simulink model "simulacao_com_referencia"  (R2020a)
settings: Solver=ode23s  StartTime=0.0  StopTime=15  FixedStep=0.001  RelTol=1e-3
values from neighbouring files (symbols this model uses):
  C_i = [C 0]    [trabalho_final.m]
  delta = mb*L*L + Ib    (= 0.00848237644)    [trabalho_final.m]
  g = 9.81    [trabalho_final.m]
  gama_i = [gama; 0]    [trabalho_final.m]
  gamah = mb*L    (= 0.039903)    [trabalho_final.m]
  K = place(phi, gama, polos)    [trabalho_final.m]
  Kec_i = inv(phi_i)*Kep_i    [trabalho_final.m]
  Nu = calc(n+1 , 1)    [trabalho_final.m]
  Nx = calc(1:n , 1)    [trabalho_final.m]
  phi_i = [phi gama; zeros(1,n) 1]    [trabalho_final.m]
  Ta = 2*pi/ws    [trabalho_final.m]
settings Model: Creator=arthu  LastModifiedBy=Acer
settings DataIOCC: LimitDataPoints=on  SaveFormat=Array  ReturnWorkspaceOutputs=off
settings OptimizationCC: LifeSpan=inf
settings DebuggingCC: SFUnexpectedBacktrackingDiag=warning  SFNoUnconditionalDefaultTransitionDiag=warning  SFExecutionAtInitializationDiag=none  ArithmeticOperatorsInVariantConditions=warning
settings HardwareCC: ProdBitPerPointer=32  ProdBitPerSizeT=32  ProdBitPerPtrDiffT=32  ProdLargestAtomicFloat=None  ProdIntDivRoundTo=Undefined  ProdEndianess=Unspecified  ProdWordSize=32  ProdHWDeviceType=32-bit Generic
settings ModelReferenceCC: PropagateSignalLabelsOutOfModel=off
settings SFSimCC: SimUseLocalCustomCode=off  CustomCodeUndefinedFunction=UseInterfaceOnly
settings RTWCC: RTWUseLocalCustomCode=off
settings CodeAppCC: StateflowObjectComments=on
settings GRTTargetCC: TargetLangStandard=C89/C90 (ANSI)
settings ConfigComp: CovMetricSettings=dw  CovHtmlReporting=on  CovSaveCumulativeToWorkspaceVar=on  CovSaveSingleToWorkspaceVar=on  CovExternalEMLEnable=off

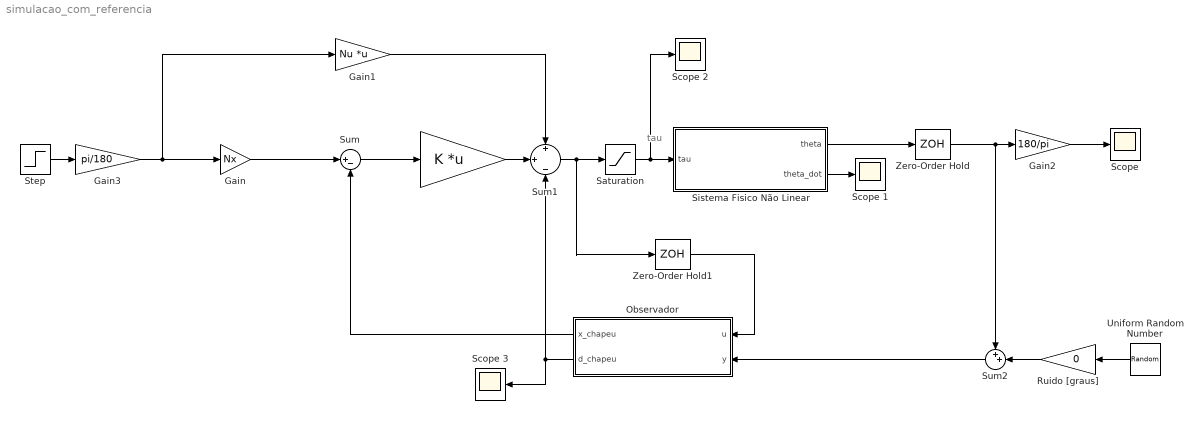
== system simulacao_com_referencia ==
  note: tau
  " " : Gain  Gain=K  Multiplication=Matrix(K*u)
  Gain : Gain  Gain=Nx
  Gain1 : Gain  Gain=Nu  Multiplication=Matrix(K*u)
  Gain2 : Gain  Gain=180/pi
  Gain3 : Gain  Gain=pi/180
  Observador : Subsystem
  Ruido [graus] : Gain  Gain=0
  "Saturation " : Saturate  UpperLimit=0.4118793  LowerLimit=-0.4118793
  Scope {,1..3} (4 alike) : Scope
  Sistema Fisico Não Linear : Subsystem
  Step : Step  After=10  SampleTime=0
  Sum : Sum  Inputs=|+-
  Sum1 : Sum  Inputs=+|+|-
  Sum2 : Sum  Inputs=++|
  "Uniform Random Number " : UniformRandomNumber  Minimum=-pi/180  Maximum=pi/180  SampleTime=Ta
  Zero-Order Hold : ZeroOrderHold  SampleTime=Ta
  Zero-Order Hold1 : ZeroOrderHold  SampleTime=Ta
  wires:
  Sistema Fisico Não Linear/1(theta) -> Zero-Order Hold/1
  Gain2/1 -> "Scope "/1
  Sistema Fisico Não Linear/2(theta_dot) -> Scope 1/1
  Observador/1(x_chapeu) -> Sum/2
  Sum/1 -> " "/1
  Gain/1 -> Sum/1
  Sum1/1 -> Zero-Order Hold1/1, "Saturation "/1
  Gain1/1 -> Sum1/1
  Step/1 -> Gain3/1
  Gain3/1 -> Gain1/1, Gain/1
  "Saturation "/1 -> Sistema Fisico Não Linear/1(tau), Scope 2/1
  Zero-Order Hold/1 -> Sum2/1, Gain2/1
  "Uniform Random Number "/1 -> Ruido [graus]/1
  Ruido [graus]/1 -> Sum2/2
  Observador/2(d_chapeu) -> Scope 3/1, Sum1/3
  " "/1 -> Sum1/2
  Zero-Order Hold1/1 -> Observador/1(u)
  Sum2/1 -> Observador/2(y)

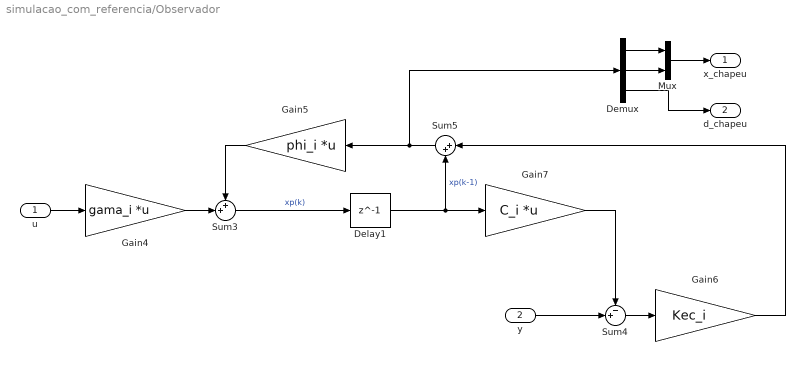
== system simulacao_com_referencia/Observador ==
  u : Inport
  y : Inport  Port=2
  Delay1 : Delay  DelayLength=1  InitialCondition=[0;0;0]
  Demux : Demux  Outputs=3
  Gain4 : Gain  Gain=gama_i  Multiplication=Matrix(K*u) (u vector)
  Gain5 : Gain  Gain=phi_i  Multiplication=Matrix(K*u) (u vector)
  Gain6 : Gain  Gain=Kec_i
  Gain7 : Gain  Gain=C_i  Multiplication=Matrix(K*u) (u vector)
  Mux : Mux  Inputs=2
  Sum3 : Sum  Inputs=++|
  Sum4 : Sum  Inputs=-+|
  Sum5 : Sum  Inputs=|++
  x_chapeu : Outport  VectorParamsAs1DForOutWhenUnconnected=off
  d_chapeu : Outport  Port=2  VectorParamsAs1DForOutWhenUnconnected=off
  wires:
  Gain6/1 -> Sum5/1
  Sum3/1 -> Delay1/1  "xp(k)"
  u/1 -> Gain4/1
  Gain4/1 -> Sum3/2
  Delay1/1 -> Gain7/1, Sum5/2  "xp(k-1)"
  Gain5/1 -> Sum3/1
  Sum4/1 -> Gain6/1
  Gain7/1 -> Sum4/1
  y/1 -> Sum4/2
  Sum5/1 -> Demux/1, Gain5/1
  Mux/1 -> x_chapeu/1
  Demux/1 -> Mux/1
  Demux/2 -> Mux/2
  Demux/3 -> d_chapeu/1

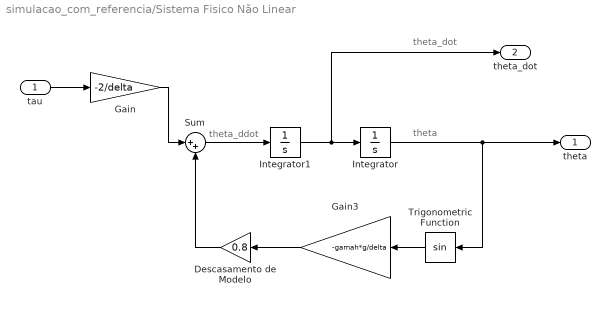
== system simulacao_com_referencia/Sistema Fisico Não Linear ==
  note: theta
  note: theta_dot
  note: theta_ddot
  tau : Inport
  Descasamento de Modelo : Gain  Gain=0.8
  Gain : Gain  Gain=-2/delta
  Gain3 : Gain  Gain=-gamah*g/delta
  Integrator : Integrator
  Integrator1 : Integrator
  Sum : Sum  Inputs=|++
  Trigonometric Function : Trigonometry
  theta : Outport
  theta_dot : Outport  Port=2
  wires:
  tau/1 -> Gain/1
  Sum/1 -> Integrator1/1
  Gain3/1 -> Descasamento de Modelo/1
  Integrator/1 -> theta/1, Trigonometric Function/1
  Trigonometric Function/1 -> Gain3/1
  Gain/1 -> Sum/1
  Integrator1/1 -> theta_dot/1, Integrator/1
  Descasamento de Modelo/1 -> Sum/2
